simulink model "walkingRobotRL3D"  (R2020b)
settings: Solver=ode23t  StartTime=0.0  StopTime=Tf  RelTol=1e-2  EnableMultiTasking=on
PreLoadFcn:
  | robotParametersRL
undefined symbols (not defined in the file): agent, ankleD_pitch_jointMAX, ankleD_pitch_jointMIN, ankleD_roll_jointMAX, ankleD_roll_jointMIN, ankleI_pitch_jointMAX, ankleI_pitch_jointMIN, ankleI_roll_jointMAX, ankleI_roll_jointMIN, getSampleTime, height_plane, hipD_pitch_jointMAX, hipD_pitch_jointMIN, hipD_roll_jointMAX, hipD_roll_jointMIN, hipI_pitch_jointMAX, hipI_pitch_jointMIN, hipI_roll_jointMAX, hipI_roll_jointMIN, init_angs_L, init_angs_R, init_height, joint_damping, joint_limit_damping, joint_limit_stiffness, joint_stiffness, kneeD_jointMAX, kneeD_jointMIN, kneeI_jointMAX, kneeI_jointMIN, lower_leg_I0, lower_leg_length, lower_leg_mass, lower_leg_x, lower_leg_y, muscle_nominal_length, p10_ankleD_roll, plane_x, plane_y, regulator_type, tau, Tf, torso_height, torso_length, torso_offset_x, torso_offset_z, torso_width, torso_x, torso_y, torso_z, Ts, upper_leg_I0, upper_leg_length, upper_leg_mass, upper_leg_x, upper_leg_y, v10_ankleD_pitch, v10_ankleD_roll, v10_ankleI_pitch, v10_ankleI_roll ... (+41)
libraries: sm_lib x222, simulink x183, nesl_utility x130, walkingRobotUtils x69, rllib x2
(part 14 of 24)

== system walkingRobotRL3D/Walking Robot (Angle based)/Antagonistic PAM Right Leg/ankleD_pitch PAM/Spring and damping model ==
  F1 : Inport
  F2 : Inport  Port=2
  P1 : Inport  Port=3
  P2 : Inport  Port=4
  Bar->kPa : Gain  Gain=100
  Bar->kPa1 : Gain  Gain=100
  Dynamic muscle 2 : Subsystem
  Dynamics muscle 1 : Subsystem
  Fplot : Scope  NumInputPorts=2
  Pplot : Scope  NumInputPorts=2
  Rplot : Scope  NumInputPorts=2
  Splot : Scope  NumInputPorts=2
  Stimation of spring coefficients : MATLAB Function  TreatAsAtomicUnit=on
  Stimation of spring coefficients1 : MATLAB Function  TreatAsAtomicUnit=on
  Unit Delay{,1..3} (4 alike) : UnitDelay  SampleTime=-1  HasFrameUpgradeWarning=on
  getDeltaXmax : Subsystem
  getDeltaXmax1 : Subsystem
  x(%)->x(m) : Gain  Gain=muscle_nominal_length/100
  x(%)->x(m)1 : Gain  Gain=muscle_nominal_length/100
  x1(m)->x1(%) : Gain  Gain=100/muscle_nominal_length
  x2(m)->x2(%) : Gain  Gain=100/muscle_nominal_length
  xplot : Scope  NumInputPorts=2
  x1 : Outport
  x2 : Outport  Port=2
  wires:
  Dynamics muscle 1/1(R1) -> Unit Delay/1, Unit Delay2/1
  Dynamic muscle 2/1(R2) -> Unit Delay1/1, Unit Delay3/1
  F1/1 -> Stimation of spring coefficients/4(F1), Fplot/1, Dynamics muscle 1/1(F1)
  Dynamic muscle 2/2(x2) -> x2(m)->x2(%)/1
  Dynamics muscle 1/2(x1) -> x1(m)->x1(%)/1
  P1/1 -> Pplot/1, Bar->kPa/1
  Bar->kPa/1 -> Stimation of spring coefficients/1(P1), getDeltaXmax/1(In1)
  P2/1 -> Pplot/2, Bar->kPa1/1
  Bar->kPa1/1 -> getDeltaXmax1/1(In1), Stimation of spring coefficients1/2(P2)
  Stimation of spring coefficients/1(S1) -> Splot/1, Dynamics muscle 1/2(S1)
  Stimation of spring coefficients1/1(S2) -> Splot/2, Dynamic muscle 2/1(S2)
  getDeltaXmax/1(dmax1) -> Stimation of spring coefficients/5(dmax1_per), x(%)->x(m)/1
  x(%)->x(m)/1 -> Stimation of spring coefficients/3(dmax1)
  getDeltaXmax1/1(dmax2) -> Stimation of spring coefficients1/5(dmax2_per), x(%)->x(m)1/1
  x(%)->x(m)1/1 -> Stimation of spring coefficients1/4(dmax2)
  x2(m)->x2(%)/1 -> xplot/2, x2/1
  x1(m)->x1(%)/1 -> xplot/1, x1/1
  F2/1 -> Stimation of spring coefficients1/1(F2), Fplot/2, Dynamic muscle 2/3(F2)
  Unit Delay/1 -> Stimation of spring coefficients1/3(Fload)
  Unit Delay1/1 -> Stimation of spring coefficients/2(Fload)
  Unit Delay2/1 -> Rplot/1, Dynamic muscle 2/2(R1)
  Unit Delay3/1 -> Rplot/2, Dynamics muscle 1/3(R2)

== system walkingRobotRL3D/Walking Robot (Angle based)/Antagonistic PAM Right Leg/ankleD_roll PAM/Spring and damping model ==
  F1 : Inport
  F2 : Inport  Port=2
  P1 : Inport  Port=3
  P2 : Inport  Port=4
  Bar->kPa : Gain  Gain=100
  Bar->kPa1 : Gain  Gain=100
  Dynamic muscle 2 : Subsystem
  Dynamics muscle 1 : Subsystem
  Fplot : Scope  NumInputPorts=2
  Pplot : Scope  NumInputPorts=2
  Rplot : Scope  NumInputPorts=2
  Splot : Scope  NumInputPorts=2
  Stimation of spring coefficients : MATLAB Function  TreatAsAtomicUnit=on
  Stimation of spring coefficients1 : MATLAB Function  TreatAsAtomicUnit=on
  Unit Delay{,1..3} (4 alike) : UnitDelay  SampleTime=-1  HasFrameUpgradeWarning=on
  getDeltaXmax : Subsystem
  getDeltaXmax1 : Subsystem
  x(%)->x(m) : Gain  Gain=muscle_nominal_length/100
  x(%)->x(m)1 : Gain  Gain=muscle_nominal_length/100
  x1(m)->x1(%) : Gain  Gain=100/muscle_nominal_length
  x2(m)->x2(%) : Gain  Gain=100/muscle_nominal_length
  xplot : Scope  NumInputPorts=2
  x1 : Outport
  x2 : Outport  Port=2
  wires:
  Dynamics muscle 1/1(R1) -> Unit Delay/1, Unit Delay2/1
  Dynamic muscle 2/1(R2) -> Unit Delay1/1, Unit Delay3/1
  F1/1 -> Stimation of spring coefficients/4(F1), Fplot/1, Dynamics muscle 1/1(F1)
  Dynamic muscle 2/2(x2) -> x2(m)->x2(%)/1
  Dynamics muscle 1/2(x1) -> x1(m)->x1(%)/1
  P1/1 -> Pplot/1, Bar->kPa/1
  Bar->kPa/1 -> Stimation of spring coefficients/1(P1), getDeltaXmax/1(In1)
  P2/1 -> Pplot/2, Bar->kPa1/1
  Bar->kPa1/1 -> getDeltaXmax1/1(In1), Stimation of spring coefficients1/2(P2)
  Stimation of spring coefficients/1(S1) -> Splot/1, Dynamics muscle 1/2(S1)
  Stimation of spring coefficients1/1(S2) -> Splot/2, Dynamic muscle 2/1(S2)
  getDeltaXmax/1(dmax1) -> Stimation of spring coefficients/5(dmax1_per), x(%)->x(m)/1
  x(%)->x(m)/1 -> Stimation of spring coefficients/3(dmax1)
  getDeltaXmax1/1(dmax2) -> Stimation of spring coefficients1/5(dmax2_per), x(%)->x(m)1/1
  x(%)->x(m)1/1 -> Stimation of spring coefficients1/4(dmax2)
  x2(m)->x2(%)/1 -> xplot/2, x2/1
  x1(m)->x1(%)/1 -> xplot/1, x1/1
  F2/1 -> Stimation of spring coefficients1/1(F2), Fplot/2, Dynamic muscle 2/3(F2)
  Unit Delay/1 -> Stimation of spring coefficients1/3(Fload)
  Unit Delay1/1 -> Stimation of spring coefficients/2(Fload)
  Unit Delay2/1 -> Rplot/1, Dynamic muscle 2/2(R1)
  Unit Delay3/1 -> Rplot/2, Dynamics muscle 1/3(R2)

== system walkingRobotRL3D/Walking Robot (Angle based)/Antagonistic PAM Right Leg/hipD_pitch PAM/Spring and damping model ==
  F1 : Inport
  F2 : Inport  Port=2
  P1 : Inport  Port=3
  P2 : Inport  Port=4
  Bar->kPa : Gain  Gain=100
  Bar->kPa1 : Gain  Gain=100
  Dynamic muscle 2 : Subsystem
  Dynamics muscle 1 : Subsystem
  Fplot : Scope  NumInputPorts=2
  Pplot : Scope  NumInputPorts=2
  Rplot : Scope  NumInputPorts=2
  Splot : Scope  NumInputPorts=2
  Stimation of spring coefficients : MATLAB Function  TreatAsAtomicUnit=on
  Stimation of spring coefficients1 : MATLAB Function  TreatAsAtomicUnit=on
  Unit Delay{,1..3} (4 alike) : UnitDelay  SampleTime=-1  HasFrameUpgradeWarning=on
  getDeltaXmax : Subsystem
  getDeltaXmax1 : Subsystem
  x(%)->x(m) : Gain  Gain=muscle_nominal_length/100
  x(%)->x(m)1 : Gain  Gain=muscle_nominal_length/100
  x1(m)->x1(%) : Gain  Gain=100/muscle_nominal_length
  x2(m)->x2(%) : Gain  Gain=100/muscle_nominal_length
  xplot : Scope  NumInputPorts=2
  x1 : Outport
  x2 : Outport  Port=2
  wires:
  Dynamics muscle 1/1(R1) -> Unit Delay/1, Unit Delay2/1
  Dynamic muscle 2/1(R2) -> Unit Delay1/1, Unit Delay3/1
  F1/1 -> Stimation of spring coefficients/4(F1), Fplot/1, Dynamics muscle 1/1(F1)
  Dynamic muscle 2/2(x2) -> x2(m)->x2(%)/1
  Dynamics muscle 1/2(x1) -> x1(m)->x1(%)/1
  P1/1 -> Pplot/1, Bar->kPa/1
  Bar->kPa/1 -> Stimation of spring coefficients/1(P1), getDeltaXmax/1(In1)
  P2/1 -> Pplot/2, Bar->kPa1/1
  Bar->kPa1/1 -> getDeltaXmax1/1(In1), Stimation of spring coefficients1/2(P2)
  Stimation of spring coefficients/1(S1) -> Splot/1, Dynamics muscle 1/2(S1)
  Stimation of spring coefficients1/1(S2) -> Splot/2, Dynamic muscle 2/1(S2)
  getDeltaXmax/1(dmax1) -> Stimation of spring coefficients/5(dmax1_per), x(%)->x(m)/1
  x(%)->x(m)/1 -> Stimation of spring coefficients/3(dmax1)
  getDeltaXmax1/1(dmax2) -> Stimation of spring coefficients1/5(dmax2_per), x(%)->x(m)1/1
  x(%)->x(m)1/1 -> Stimation of spring coefficients1/4(dmax2)
  x2(m)->x2(%)/1 -> xplot/2, x2/1
  x1(m)->x1(%)/1 -> xplot/1, x1/1
  F2/1 -> Stimation of spring coefficients1/1(F2), Fplot/2, Dynamic muscle 2/3(F2)
  Unit Delay/1 -> Stimation of spring coefficients1/3(Fload)
  Unit Delay1/1 -> Stimation of spring coefficients/2(Fload)
  Unit Delay2/1 -> Rplot/1, Dynamic muscle 2/2(R1)
  Unit Delay3/1 -> Rplot/2, Dynamics muscle 1/3(R2)

== system walkingRobotRL3D/Walking Robot (Angle based)/Antagonistic PAM Right Leg/hipD_roll PAM/Spring and damping model ==
  F1 : Inport
  F2 : Inport  Port=2
  P1 : Inport  Port=3
  P2 : Inport  Port=4
  Bar->kPa : Gain  Gain=100
  Bar->kPa1 : Gain  Gain=100
  Dynamic muscle 2 : Subsystem
  Dynamics muscle 1 : Subsystem
  Fplot : Scope  NumInputPorts=2
  Pplot : Scope  NumInputPorts=2
  Rplot : Scope  NumInputPorts=2
  Splot : Scope  NumInputPorts=2
  Stimation of spring coefficients : MATLAB Function  TreatAsAtomicUnit=on
  Stimation of spring coefficients1 : MATLAB Function  TreatAsAtomicUnit=on
  Unit Delay{,1..3} (4 alike) : UnitDelay  SampleTime=-1  HasFrameUpgradeWarning=on
  getDeltaXmax : Subsystem
  getDeltaXmax1 : Subsystem
  x(%)->x(m) : Gain  Gain=muscle_nominal_length/100
  x(%)->x(m)1 : Gain  Gain=muscle_nominal_length/100
  x1(m)->x1(%) : Gain  Gain=100/muscle_nominal_length
  x2(m)->x2(%) : Gain  Gain=100/muscle_nominal_length
  xplot : Scope  NumInputPorts=2
  x1 : Outport
  x2 : Outport  Port=2
  wires:
  Dynamics muscle 1/1(R1) -> Unit Delay/1, Unit Delay2/1
  Dynamic muscle 2/1(R2) -> Unit Delay1/1, Unit Delay3/1
  F1/1 -> Stimation of spring coefficients/4(F1), Fplot/1, Dynamics muscle 1/1(F1)
  Dynamic muscle 2/2(x2) -> x2(m)->x2(%)/1
  Dynamics muscle 1/2(x1) -> x1(m)->x1(%)/1
  P1/1 -> Pplot/1, Bar->kPa/1
  Bar->kPa/1 -> Stimation of spring coefficients/1(P1), getDeltaXmax/1(In1)
  P2/1 -> Pplot/2, Bar->kPa1/1
  Bar->kPa1/1 -> getDeltaXmax1/1(In1), Stimation of spring coefficients1/2(P2)
  Stimation of spring coefficients/1(S1) -> Splot/1, Dynamics muscle 1/2(S1)
  Stimation of spring coefficients1/1(S2) -> Splot/2, Dynamic muscle 2/1(S2)
  getDeltaXmax/1(dmax1) -> Stimation of spring coefficients/5(dmax1_per), x(%)->x(m)/1
  x(%)->x(m)/1 -> Stimation of spring coefficients/3(dmax1)
  getDeltaXmax1/1(dmax2) -> Stimation of spring coefficients1/5(dmax2_per), x(%)->x(m)1/1
  x(%)->x(m)1/1 -> Stimation of spring coefficients1/4(dmax2)
  x2(m)->x2(%)/1 -> xplot/2, x2/1
  x1(m)->x1(%)/1 -> xplot/1, x1/1
  F2/1 -> Stimation of spring coefficients1/1(F2), Fplot/2, Dynamic muscle 2/3(F2)
  Unit Delay/1 -> Stimation of spring coefficients1/3(Fload)
  Unit Delay1/1 -> Stimation of spring coefficients/2(Fload)
  Unit Delay2/1 -> Rplot/1, Dynamic muscle 2/2(R1)
  Unit Delay3/1 -> Rplot/2, Dynamics muscle 1/3(R2)

== system walkingRobotRL3D/Walking Robot (Angle based)/Antagonistic PAM Right Leg/kneeD PAM/Spring and damping model ==
  F1 : Inport
  F2 : Inport  Port=2
  P1 : Inport  Port=3
  P2 : Inport  Port=4
  Bar->kPa : Gain  Gain=100
  Bar->kPa1 : Gain  Gain=100
  Dynamic muscle 2 : Subsystem
  Dynamics muscle 1 : Subsystem
  Fplot : Scope  NumInputPorts=2
  Pplot : Scope  NumInputPorts=2
  Rplot : Scope  NumInputPorts=2
  Splot : Scope  NumInputPorts=2
  Stimation of spring coefficients : MATLAB Function  TreatAsAtomicUnit=on
  Stimation of spring coefficients1 : MATLAB Function  TreatAsAtomicUnit=on
  Unit Delay{,1..3} (4 alike) : UnitDelay  SampleTime=-1  HasFrameUpgradeWarning=on
  getDeltaXmax : Subsystem
  getDeltaXmax1 : Subsystem
  x(%)->x(m) : Gain  Gain=muscle_nominal_length/100
  x(%)->x(m)1 : Gain  Gain=muscle_nominal_length/100
  x1(m)->x1(%) : Gain  Gain=100/muscle_nominal_length
  x2(m)->x2(%) : Gain  Gain=100/muscle_nominal_length
  xplot : Scope  NumInputPorts=2
  x1 : Outport
  x2 : Outport  Port=2
  wires:
  Dynamics muscle 1/1(R1) -> Unit Delay/1, Unit Delay2/1
  Dynamic muscle 2/1(R2) -> Unit Delay1/1, Unit Delay3/1
  F1/1 -> Stimation of spring coefficients/4(F1), Fplot/1, Dynamics muscle 1/1(F1)
  Dynamic muscle 2/2(x2) -> x2(m)->x2(%)/1
  Dynamics muscle 1/2(x1) -> x1(m)->x1(%)/1
  P1/1 -> Pplot/1, Bar->kPa/1
  Bar->kPa/1 -> Stimation of spring coefficients/1(P1), getDeltaXmax/1(In1)
  P2/1 -> Pplot/2, Bar->kPa1/1
  Bar->kPa1/1 -> getDeltaXmax1/1(In1), Stimation of spring coefficients1/2(P2)
  Stimation of spring coefficients/1(S1) -> Splot/1, Dynamics muscle 1/2(S1)
  Stimation of spring coefficients1/1(S2) -> Splot/2, Dynamic muscle 2/1(S2)
  getDeltaXmax/1(dmax1) -> Stimation of spring coefficients/5(dmax1_per), x(%)->x(m)/1
  x(%)->x(m)/1 -> Stimation of spring coefficients/3(dmax1)
  getDeltaXmax1/1(dmax2) -> Stimation of spring coefficients1/5(dmax2_per), x(%)->x(m)1/1
  x(%)->x(m)1/1 -> Stimation of spring coefficients1/4(dmax2)
  x2(m)->x2(%)/1 -> xplot/2, x2/1
  x1(m)->x1(%)/1 -> xplot/1, x1/1
  F2/1 -> Stimation of spring coefficients1/1(F2), Fplot/2, Dynamic muscle 2/3(F2)
  Unit Delay/1 -> Stimation of spring coefficients1/3(Fload)
  Unit Delay1/1 -> Stimation of spring coefficients/2(Fload)
  Unit Delay2/1 -> Rplot/1, Dynamic muscle 2/2(R1)
  Unit Delay3/1 -> Rplot/2, Dynamics muscle 1/3(R2)

== system walkingRobotRL3D/Walking Robot (Angle based)/Dynamic model of antagonistic PAM actuators/Spring//Damping (Muscles 1)/Get_delta_xmax1 ==
  P1 : Inport
  Bar->kPa : Product
  Constant : Constant  Value=100
  Demux : Demux  Outputs=10
  Mux : Mux  Inputs=10
  Mux1 : Mux  Inputs=10
  getDeltaXmax : Subsystem
  getDeltaXmax1 : Subsystem
  getDeltaXmax2 : Subsystem
  getDeltaXmax3 : Subsystem
  getDeltaXmax4 : Subsystem
  getDeltaXmax5 : Subsystem
  getDeltaXmax6 : Subsystem
  getDeltaXmax7 : Subsystem
  getDeltaXmax8 : Subsystem
  getDeltaXmax9 : Subsystem
  xmax_muscles1 : Outport
  delta_xmax_muscles1_per : Outport  Port=2
  wires:
  P1/1 -> Bar->kPa/2
  Bar->kPa/1 -> Demux/1
  Constant/1 -> Bar->kPa/1
  Mux/1 -> xmax_muscles1/1
  Demux/1 -> getDeltaXmax/1(In1)
  getDeltaXmax/1(Out1) -> Mux/1
  Mux1/1 -> delta_xmax_muscles1_per/1
  Demux/2 -> getDeltaXmax1/1(In1)
  Demux/3 -> getDeltaXmax2/1(In1)
  Demux/4 -> getDeltaXmax3/1(In1)
  Demux/5 -> getDeltaXmax4/1(In1)
  Demux/6 -> getDeltaXmax5/1(In1)
  Demux/7 -> getDeltaXmax6/1(In1)
  Demux/8 -> getDeltaXmax7/1(In1)
  Demux/9 -> getDeltaXmax8/1(In1)
  getDeltaXmax1/1(Out1) -> Mux/2
  getDeltaXmax2/1(Out1) -> Mux/3
  getDeltaXmax3/1(Out1) -> Mux/4
  getDeltaXmax4/1(Out1) -> Mux/5
  getDeltaXmax5/1(Out1) -> Mux/6
  getDeltaXmax6/1(Out1) -> Mux/7
  getDeltaXmax7/1(Out1) -> Mux/8
  getDeltaXmax8/1(Out1) -> Mux/9
  getDeltaXmax9/1(Out1) -> Mux/10
  getDeltaXmax/2(Out2) -> Mux1/1
  getDeltaXmax1/2(Out2) -> Mux1/2
  getDeltaXmax2/2(Out2) -> Mux1/3
  getDeltaXmax3/2(Out2) -> Mux1/4
  getDeltaXmax4/2(Out2) -> Mux1/5
  getDeltaXmax5/2(Out2) -> Mux1/6
  getDeltaXmax6/2(Out2) -> Mux1/7
  getDeltaXmax7/2(Out2) -> Mux1/8
  getDeltaXmax8/2(Out2) -> Mux1/9
  Demux/10 -> getDeltaXmax9/1(In1)
  getDeltaXmax9/2(Out2) -> Mux1/10

== system walkingRobotRL3D/Walking Robot (Angle based)/Dynamic model of antagonistic PAM actuators/Spring//Damping (Muscles 1)/Get_x1_ankleD_pitch ==
  F1_ankleD_pitchl : Inport
  F2_ankleD_pitch : Inport  Port=2
  S_coef : Inport  Port=3
  Add : Sum  Inputs=+--
  Constant : Constant  Value=tau
  Constant1 : Constant
  Constant2 : Constant  Commented=on  Value=-3.9322
  D_coef : Product
  Divide : Product  Inputs=*/
  IC : InitialCondition  Commented=through  Value=10000
  Integrator : Integrator  InitialCondition=x10_ankleD_pitch
  To Workspace : ToWorkspace  VariableName=S1_ankleD_pitch  SaveFormat=Timeseries  SampleTime=-1
  To Workspace1 : ToWorkspace  VariableName=D1_ankleD_pitch  SaveFormat=Timeseries  SampleTime=-1
  x./D : Product
  xS : Product
  x1_ankleD_pitch : Outport
  wires:
  xS/1 -> Add/3
  x./D/1 -> Integrator/1
  Constant/1 -> D_coef/1
  Divide/1 -> x./D/1
  Constant1/1 -> Divide/1
  D_coef/1 -> To Workspace1/1, Divide/2
  Integrator/1 -> x1_ankleD_pitch/1, xS/1
  IC/1 -> xS/2, To Workspace/1, D_coef/2
  F1_ankleD_pitchl/1 -> Add/1
  F2_ankleD_pitch/1 -> Add/2
  S_coef/1 -> IC/1
  Add/1 -> x./D/2

== system walkingRobotRL3D/Walking Robot (Angle based)/Dynamic model of antagonistic PAM actuators/Spring//Damping (Muscles 1)/Get_x1_ankleD_roll ==
  F1_ankleD_roll : Inport
  F2_ankleD_roll : Inport  Port=2
  S_coef : Inport  Port=3
  Add : Sum  Inputs=+--
  Constant : Constant  Value=tau
  Constant1 : Constant
  Constant2 : Constant  Commented=on  Value=-3.9322
  D_coef : Product
  Divide : Product  Inputs=*/
  IC : InitialCondition  Commented=through  Value=10000
  Integrator : Integrator  InitialCondition=x10_ankleD_roll
  To Workspace : ToWorkspace  VariableName=S1_ankleD_roll  SaveFormat=Timeseries  SampleTime=-1
  To Workspace1 : ToWorkspace  VariableName=D1_ankleD_roll  SaveFormat=Timeseries  SampleTime=-1
  x./D : Product
  xS : Product
  x1_ankleD_roll : Outport
  wires:
  xS/1 -> Add/3
  x./D/1 -> Integrator/1
  Constant/1 -> D_coef/1
  Divide/1 -> x./D/1
  Constant1/1 -> Divide/1
  D_coef/1 -> To Workspace1/1, Divide/2
  Integrator/1 -> x1_ankleD_roll/1, xS/1
  IC/1 -> xS/2, To Workspace/1, D_coef/2
  F1_ankleD_roll/1 -> Add/1
  F2_ankleD_roll/1 -> Add/2
  Add/1 -> x./D/2
  S_coef/1 -> IC/1

== system walkingRobotRL3D/Walking Robot (Angle based)/Dynamic model of antagonistic PAM actuators/Spring//Damping (Muscles 1)/Get_x1_ankleI_pitch ==
  F1_ankleI_pitch : Inport
  F2_ankleI_pitch : Inport  Port=2
  S_coef : Inport  Port=3
  Add : Sum  Inputs=+--
  Constant : Constant  Value=tau
  Constant1 : Constant
  D_coef : Product
  Divide : Product  Inputs=*/
  Integrator : Integrator  InitialCondition=x10_ankleI_pitch
  x./D : Product
  xS : Product
  x1_ankleI_pitch : Outport
  wires:
  xS/1 -> Add/3
  Add/1 -> x./D/2
  F1_ankleI_pitch/1 -> Add/1
  F2_ankleI_pitch/1 -> Add/2
  Integrator/1 -> x1_ankleI_pitch/1, xS/1
  S_coef/1 -> D_coef/2, xS/2
  x./D/1 -> Integrator/1
  Constant/1 -> D_coef/1
  Divide/1 -> x./D/1
  Constant1/1 -> Divide/1
  D_coef/1 -> Divide/2

== system walkingRobotRL3D/Walking Robot (Angle based)/Dynamic model of antagonistic PAM actuators/Spring//Damping (Muscles 1)/Get_x1_ankleI_roll ==
  F1_ankleI_roll : Inport
  F2_ankleI_roll : Inport  Port=2
  S_coef : Inport  Port=3
  Add : Sum  Inputs=+--
  Constant : Constant  Value=tau
  Constant1 : Constant
  D_coef : Product
  Divide : Product  Inputs=*/
  Integrator : Integrator  InitialCondition=x10_ankleI_roll
  x./D : Product
  xS : Product
  x1_ankleI_roll : Outport
  wires:
  xS/1 -> Add/3
  Add/1 -> x./D/2
  F1_ankleI_roll/1 -> Add/1
  F2_ankleI_roll/1 -> Add/2
  Integrator/1 -> x1_ankleI_roll/1, xS/1
  S_coef/1 -> D_coef/2, xS/2
  x./D/1 -> Integrator/1
  Constant/1 -> D_coef/1
  Divide/1 -> x./D/1
  Constant1/1 -> Divide/1
  D_coef/1 -> Divide/2

== system walkingRobotRL3D/Walking Robot (Angle based)/Dynamic model of antagonistic PAM actuators/Spring//Damping (Muscles 1)/Get_x1_hipD_pitch ==
  F1_hipD_pitch : Inport
  F2_hipD_pitch : Inport  Port=2
  S_coef : Inport  Port=3
  Add : Sum  Inputs=+--
  Constant : Constant  Value=tau
  Constant1 : Constant
  D_coef : Product
  Divide : Product  Inputs=*/
  Integrator : Integrator  InitialCondition=x10_hipD_pitch
  x./D : Product
  xS : Product
  x1_hipD_pitch : Outport
  wires:
  xS/1 -> Add/3
  Add/1 -> x./D/2
  F1_hipD_pitch/1 -> Add/1
  F2_hipD_pitch/1 -> Add/2
  Integrator/1 -> x1_hipD_pitch/1, xS/1
  S_coef/1 -> D_coef/2, xS/2
  x./D/1 -> Integrator/1
  Constant/1 -> D_coef/1
  Divide/1 -> x./D/1
  Constant1/1 -> Divide/1
  D_coef/1 -> Divide/2

== system walkingRobotRL3D/Walking Robot (Angle based)/Dynamic model of antagonistic PAM actuators/Spring//Damping (Muscles 1)/Get_x1_hipD_roll ==
  F1_hipD_roll : Inport
  F2_hipD_roll : Inport  Port=2
  S_coef : Inport  Port=3
  Add : Sum  Inputs=+--
  Constant : Constant  Value=tau
  Constant1 : Constant
  D_coef : Product
  Divide : Product  Inputs=*/
  Integrator : Integrator  InitialCondition=x10_hipD_roll
  x./D : Product
  xS : Product
  x1_hipD_roll : Outport
  wires:
  xS/1 -> Add/3
  Add/1 -> x./D/2
  F1_hipD_roll/1 -> Add/1
  F2_hipD_roll/1 -> Add/2
  Integrator/1 -> x1_hipD_roll/1, xS/1
  S_coef/1 -> D_coef/2, xS/2
  x./D/1 -> Integrator/1
  Constant/1 -> D_coef/1
  Divide/1 -> x./D/1
  Constant1/1 -> Divide/1
  D_coef/1 -> Divide/2

== system walkingRobotRL3D/Walking Robot (Angle based)/Dynamic model of antagonistic PAM actuators/Spring//Damping (Muscles 1)/Get_x1_hipI_pitch ==
  F1_hipI_pitch : Inport
  F2_hipI_pitch : Inport  Port=2
  S_coef : Inport  Port=3
  Add : Sum  Inputs=+--
  Constant : Constant  Value=tau
  Constant1 : Constant
  D_coef : Product
  Divide : Product  Inputs=*/
  Integrator : Integrator  InitialCondition=x10_hipI_pitch
  Relay : Relay  Commented=through  OnSwitchValue=28.12*muscle_nominal_length/100  OffSwitchValue=0  OnOutputValue=28.12*muscle_nominal_length/100
  x./D : Product
  xS : Product
  x1_hipI_pitch : Outport
  wires:
  xS/1 -> Add/3
  Add/1 -> x./D/2
  F1_hipI_pitch/1 -> Add/1
  F2_hipI_pitch/1 -> Add/2
  S_coef/1 -> D_coef/2, xS/2
  x./D/1 -> Integrator/1
  Constant/1 -> D_coef/1
  Divide/1 -> x./D/1
  Constant1/1 -> Divide/1
  D_coef/1 -> Divide/2
  Integrator/1 -> Relay/1
  Relay/1 -> xS/1, x1_hipI_pitch/1

== system walkingRobotRL3D/Walking Robot (Angle based)/Dynamic model of antagonistic PAM actuators/Spring//Damping (Muscles 1)/Get_x1_hipI_roll ==
  F1_hipI_roll : Inport
  F2_hipI_roll : Inport  Port=2
  S_coef : Inport  Port=3
  Add : Sum  Inputs=+--
  Constant : Constant  Value=tau
  Constant1 : Constant
  D_coef : Product
  Divide : Product  Inputs=*/
  Integrator : Integrator  InitialCondition=x10_hipI_roll
  x./D : Product
  xS : Product
  x1_hipI_roll : Outport
  wires:
  xS/1 -> Add/3
  Add/1 -> x./D/2
  F1_hipI_roll/1 -> Add/1
  F2_hipI_roll/1 -> Add/2
  Integrator/1 -> x1_hipI_roll/1, xS/1
  S_coef/1 -> D_coef/2, xS/2
  x./D/1 -> Integrator/1
  Constant/1 -> D_coef/1
  Divide/1 -> x./D/1
  Constant1/1 -> Divide/1
  D_coef/1 -> Divide/2

== system walkingRobotRL3D/Walking Robot (Angle based)/Dynamic model of antagonistic PAM actuators/Spring//Damping (Muscles 1)/Get_x1_kneeD_1 ==
  F1_kneeD : Inport
  F2_kneeD : Inport  Port=2
  S_coef : Inport  Port=3
  Add : Sum  Inputs=++-
  Constant : Constant  Value=tau
  Constant1 : Constant
  D_coef : Product
  Divide : Product  Inputs=*/
  Integrator : Integrator  InitialCondition=x10_kneeD
  x./D : Product
  xS : Product
  x1_kneeD : Outport
  wires:
  xS/1 -> Add/3
  Add/1 -> x./D/2
  F1_kneeD/1 -> Add/1
  F2_kneeD/1 -> Add/2
  Integrator/1 -> x1_kneeD/1, xS/1
  S_coef/1 -> D_coef/2, xS/2
  x./D/1 -> Integrator/1
  Constant/1 -> D_coef/1
  Divide/1 -> x./D/1
  Constant1/1 -> Divide/1
  D_coef/1 -> Divide/2

== system walkingRobotRL3D/Walking Robot (Angle based)/Dynamic model of antagonistic PAM actuators/Spring//Damping (Muscles 1)/Get_x1_kneeI ==
  F1_kneeI : Inport
  F2_kneeI : Inport  Port=2
  S_coef : Inport  Port=3
  Abs2 : Abs
  Add : Sum  Inputs=++-
  Constant : Constant  Value=tau
  Constant1 : Constant
  D_coef : Product
  Divide : Product  Inputs=*/
  Integrator : Integrator  InitialCondition=x10_kneeI
  x./D : Product
  xS : Product
  x1_kneeI : Outport
  wires:
  F1_kneeI/1 -> Add/1
  Integrator/1 -> x1_kneeI/1, xS/1
  S_coef/1 -> Abs2/1
  x./D/1 -> Integrator/1
  Constant/1 -> D_coef/1
  Divide/1 -> x./D/1
  Constant1/1 -> Divide/1
  D_coef/1 -> Divide/2
  Abs2/1 -> xS/2, D_coef/2
  xS/1 -> Add/3
  F2_kneeI/1 -> Add/2
  Add/1 -> x./D/2

== system walkingRobotRL3D/Walking Robot (Angle based)/Dynamic model of antagonistic PAM actuators/Spring//Damping (Muscles 2)/Get_x2_ankleD_pitch ==
  F1_ankleD_pitch : Inport
  F2_ankleD_pitch : Inport  Port=2
  S2_coef : Inport  Port=3
  Add : Sum  Inputs=-+-
  Constant : Constant  Value=tau
  Constant1 : Constant
  Constant2 : Constant  Commented=on  Value=3.9338
  D_coef : Product
  Divide : Product  Inputs=*/
  IC : InitialCondition  Commented=through  Value=3.9338
  Integrator : Integrator  InitialCondition=x20_ankleD_pitch
  To Workspace : ToWorkspace  VariableName=S2_ankleD_pitch  SaveFormat=Timeseries  SampleTime=-1
  x./D : Product
  xS : Product
  x2_ankleD_pitch : Outport
  wires:
  xS/1 -> Add/3
  Add/1 -> x./D/2
  F1_ankleD_pitch/1 -> Add/1
  F2_ankleD_pitch/1 -> Add/2
  Integrator/1 -> x2_ankleD_pitch/1, xS/1
  x./D/1 -> Integrator/1
  Constant/1 -> D_coef/1
  Divide/1 -> x./D/1
  Constant1/1 -> Divide/1
  IC/1 -> To Workspace/1, D_coef/2, xS/2
  D_coef/1 -> Divide/2
  S2_coef/1 -> IC/1

== system walkingRobotRL3D/Walking Robot (Angle based)/Dynamic model of antagonistic PAM actuators/Spring//Damping (Muscles 2)/Get_x2_ankleD_roll ==
  F1_ankleD_roll : Inport
  F2_ankleD_roll : Inport  Port=2
  S2_coef : Inport  Port=3
  Add : Sum  Inputs=-+-
  Constant : Constant  Value=tau
  Constant1 : Constant
  Constant2 : Constant  Commented=on  Value=3.9338
  D_coef : Product
  Divide : Product  Inputs=*/
  IC : InitialCondition  Commented=through  Value=3.9338
  Integrator : Integrator  InitialCondition=x20_ankleD_roll
  To Workspace : ToWorkspace  VariableName=S2_ankleD_roll  SaveFormat=Timeseries  SampleTime=-1
  x./D : Product
  xS : Product
  x2_ankleD_roll : Outport
  wires:
  xS/1 -> Add/3
  Add/1 -> x./D/2
  F1_ankleD_roll/1 -> Add/1
  F2_ankleD_roll/1 -> Add/2
  Integrator/1 -> x2_ankleD_roll/1, xS/1
  x./D/1 -> Integrator/1
  Constant/1 -> D_coef/1
  Divide/1 -> x./D/1
  Constant1/1 -> Divide/1
  IC/1 -> To Workspace/1, D_coef/2, xS/2
  D_coef/1 -> Divide/2
  S2_coef/1 -> IC/1

== system walkingRobotRL3D/Walking Robot (Angle based)/Dynamic model of antagonistic PAM actuators/Spring//Damping (Muscles 2)/Get_x2_ankleI_pitch ==
  F1_ankleI_pitch : Inport
  F2_ankleI_pitch : Inport  Port=2
  S2_coef : Inport  Port=3
  Add : Sum  Inputs=-+-
  Constant : Constant  Value=tau
  Constant1 : Constant
  D_coef : Product
  Divide : Product  Inputs=*/
  Integrator : Integrator  InitialCondition=x20_ankleI_pitch
  x./D : Product
  xS : Product
  x2_ankleI_pitch : Outport
  wires:
  xS/1 -> Add/3
  Add/1 -> x./D/2
  F1_ankleI_pitch/1 -> Add/1
  F2_ankleI_pitch/1 -> Add/2
  Integrator/1 -> x2_ankleI_pitch/1, xS/1
  S2_coef/1 -> D_coef/2, xS/2
  x./D/1 -> Integrator/1
  Constant/1 -> D_coef/1
  Divide/1 -> x./D/1
  Constant1/1 -> Divide/1
  D_coef/1 -> Divide/2

== system walkingRobotRL3D/Walking Robot (Angle based)/Dynamic model of antagonistic PAM actuators/Spring//Damping (Muscles 2)/Get_x2_ankleI_roll ==
  F1_ankleI_roll : Inport
  F2_ankleI_roll : Inport  Port=2
  S2_coef : Inport  Port=3
  Add : Sum  Inputs=-+-
  Constant : Constant  Value=tau
  Constant1 : Constant
  D_coef : Product
  Divide : Product  Inputs=*/
  Integrator : Integrator  InitialCondition=x20_ankleI_roll
  x./D : Product
  xS : Product
  x2_ankleI_roll : Outport
  wires:
  xS/1 -> Add/3
  Add/1 -> x./D/2
  F1_ankleI_roll/1 -> Add/1
  F2_ankleI_roll/1 -> Add/2
  Integrator/1 -> x2_ankleI_roll/1, xS/1
  S2_coef/1 -> D_coef/2, xS/2
  x./D/1 -> Integrator/1
  Constant/1 -> D_coef/1
  Divide/1 -> x./D/1
  Constant1/1 -> Divide/1
  D_coef/1 -> Divide/2

== system walkingRobotRL3D/Walking Robot (Angle based)/Dynamic model of antagonistic PAM actuators/Spring//Damping (Muscles 2)/Get_x2_hipD_pitch ==
  F1_hipD_pitch : Inport
  F2_hipD_pitch : Inport  Port=2
  S2_coef : Inport  Port=3
  Add : Sum  Inputs=-+-
  Constant : Constant  Value=tau
  Constant1 : Constant
  D_coef : Product
  Divide : Product  Inputs=*/
  Integrator : Integrator  InitialCondition=x20_hipD_pitch
  x./D : Product
  xS : Product
  x2_hipD_pitch : Outport
  wires:
  xS/1 -> Add/3
  Add/1 -> x./D/2
  F1_hipD_pitch/1 -> Add/1
  F2_hipD_pitch/1 -> Add/2
  Integrator/1 -> x2_hipD_pitch/1, xS/1
  S2_coef/1 -> D_coef/2, xS/2
  x./D/1 -> Integrator/1
  Constant/1 -> D_coef/1
  Divide/1 -> x./D/1
  Constant1/1 -> Divide/1
  D_coef/1 -> Divide/2

== system walkingRobotRL3D/Walking Robot (Angle based)/Dynamic model of antagonistic PAM actuators/Spring//Damping (Muscles 2)/Get_x2_hipD_roll ==
  F1_hipD_roll : Inport
  F2_hipD_roll : Inport  Port=2
  S2_coef : Inport  Port=3
  Add : Sum  Inputs=-+-
  Constant : Constant  Value=tau
  Constant1 : Constant
  D_coef : Product
  Divide : Product  Inputs=*/
  Integrator : Integrator  InitialCondition=x20_hipD_roll
  x./D : Product
  xS : Product
  x2_hipD_roll : Outport
  wires:
  xS/1 -> Add/3
  Add/1 -> x./D/2
  F1_hipD_roll/1 -> Add/1
  F2_hipD_roll/1 -> Add/2
  Integrator/1 -> x2_hipD_roll/1, xS/1
  S2_coef/1 -> D_coef/2, xS/2
  x./D/1 -> Integrator/1
  Constant/1 -> D_coef/1
  Divide/1 -> x./D/1
  Constant1/1 -> Divide/1
  D_coef/1 -> Divide/2

== system walkingRobotRL3D/Walking Robot (Angle based)/Dynamic model of antagonistic PAM actuators/Spring//Damping (Muscles 2)/Get_x2_hipI_pitch ==
  F1_hipI_pitch : Inport
  F2_hipI_pitch : Inport  Port=2
  S2_coef : Inport  Port=3
  Add : Sum  Inputs=-+-
  Constant : Constant  Value=tau
  Constant1 : Constant
  D_coef : Product
  Divide : Product  Inputs=*/
  Integrator : Integrator  InitialCondition=x20_hipI_pitch
  Relay : Relay  Commented=through  OnSwitchValue=28.12*muscle_nominal_length/100  OffSwitchValue=0  OnOutputValue=28.12*muscle_nominal_length/100
  x./D : Product
  xS : Product
  x2_hipI_pitch : Outport
  wires:
  xS/1 -> Add/3
  Add/1 -> x./D/2
  F1_hipI_pitch/1 -> Add/1
  F2_hipI_pitch/1 -> Add/2
  Integrator/1 -> Relay/1
  S2_coef/1 -> D_coef/2, xS/2
  x./D/1 -> Integrator/1
  Constant/1 -> D_coef/1
  Divide/1 -> x./D/1
  Constant1/1 -> Divide/1
  D_coef/1 -> Divide/2
  Relay/1 -> x2_hipI_pitch/1, xS/1

== system walkingRobotRL3D/Walking Robot (Angle based)/Dynamic model of antagonistic PAM actuators/Spring//Damping (Muscles 2)/Get_x2_hipI_roll ==
  F1_hipI_roll : Inport
  F2_hipI_roll : Inport  Port=2
  S2_coef : Inport  Port=3
  Add : Sum  Inputs=-+-
  Constant : Constant  Value=tau
  Constant1 : Constant
  D_coef : Product
  Divide : Product  Inputs=*/
  Integrator : Integrator  InitialCondition=x20_hipI_roll
  x./D : Product
  xS : Product
  x2_hipI_roll : Outport
  wires:
  xS/1 -> Add/3
  Add/1 -> x./D/2
  F1_hipI_roll/1 -> Add/1
  F2_hipI_roll/1 -> Add/2
  Integrator/1 -> x2_hipI_roll/1, xS/1
  S2_coef/1 -> D_coef/2, xS/2
  x./D/1 -> Integrator/1
  Constant/1 -> D_coef/1
  Divide/1 -> x./D/1
  Constant1/1 -> Divide/1
  D_coef/1 -> Divide/2

== system walkingRobotRL3D/Walking Robot (Angle based)/Dynamic model of antagonistic PAM actuators/Spring//Damping (Muscles 2)/Get_x2_kneeD ==
  F1_kneeD : Inport
  F2_kneeI : Inport  Port=2
  S2_coef : Inport  Port=3
  Add : Sum  Inputs=-+-
  Constant : Constant  Value=tau
  Constant1 : Constant
  D_coef : Product
  Divide : Product  Inputs=*/
  Integrator : Integrator  InitialCondition=x20_kneeD
  x./D : Product
  xS : Product
  x2_kneeD : Outport
  wires:
  xS/1 -> Add/3
  Add/1 -> x./D/2
  F1_kneeD/1 -> Add/1
  F2_kneeI/1 -> Add/2
  Integrator/1 -> x2_kneeD/1, xS/1
  S2_coef/1 -> D_coef/2, xS/2
  x./D/1 -> Integrator/1
  Constant/1 -> D_coef/1
  Divide/1 -> x./D/1
  Constant1/1 -> Divide/1
  D_coef/1 -> Divide/2

== system walkingRobotRL3D/Walking Robot (Angle based)/Dynamic model of antagonistic PAM actuators/Spring//Damping (Muscles 2)/Get_x2_kneeI ==
  F1_kneeI : Inport
  F2_kneeI : Inport  Port=2
  S2_coef : Inport  Port=3
  Add : Sum  Inputs=++-
  Constant : Constant  Value=tau
  Constant1 : Constant
  D_coef : Product
  Divide : Product  Inputs=*/
  Integrator : Integrator  InitialCondition=x20_kneeI
  x./D : Product
  xS : Product
  x2_kneeI : Outport
  wires:
  xS/1 -> Add/3
  Add/1 -> x./D/2
  F1_kneeI/1 -> Add/1
  F2_kneeI/1 -> Add/2
  Integrator/1 -> x2_kneeI/1, xS/1
  S2_coef/1 -> D_coef/2, xS/2
  x./D/1 -> Integrator/1
  Constant/1 -> D_coef/1
  Divide/1 -> x./D/1
  Constant1/1 -> Divide/1
  D_coef/1 -> Divide/2

== system walkingRobotRL3D/Walking Robot (Angle based)/Dynamic model of antagonistic PAM actuators/Spring//Damping (Muscles 2)/Getxmax2 ==
  P2 : Inport
  Get_delta_xmax1 : Subsystem
  delta_xmax_muscles2 : Outport
  delta_xmax_muscles2_per : Outport  Port=2
  wires:
  P2/1 -> Get_delta_xmax1/1(P2)
  Get_delta_xmax1/1(delta_xmax_muscles2) -> delta_xmax_muscles2/1
  Get_delta_xmax1/2(delta_xmax_muscles2_per) -> delta_xmax_muscles2_per/1

== system walkingRobotRL3D/Walking Robot1/Dynamic model of antagonistic PAM actuators/Spring//Damping (Muscles 1)/Get_x1_ankleD_pitch ==
  F1_ankleD_pitchl : Inport
  F2_ankleD_pitch : Inport  Port=2
  S_coef : Inport  Port=3
  Add : Sum  Inputs=+--
  Constant : Constant  Value=tau
  Constant1 : Constant
  Constant2 : Constant  Commented=on  Value=-3.9322
  D_coef : Product
  Divide : Product  Inputs=*/
  IC : InitialCondition  Commented=through  Value=-3.9322
  Integrator : Integrator  InitialCondition=x10_ankleD_pitch
  x./D : Product
  xS : Product
  x1_ankleD_pitch : Outport
  wires:
  xS/1 -> Add/3
  x./D/1 -> Integrator/1
  Constant/1 -> D_coef/1
  Divide/1 -> x./D/1
  Constant1/1 -> Divide/1
  D_coef/1 -> Divide/2
  Integrator/1 -> x1_ankleD_pitch/1, xS/1
  IC/1 -> xS/2, D_coef/2
  F1_ankleD_pitchl/1 -> Add/1
  F2_ankleD_pitch/1 -> Add/2
  S_coef/1 -> IC/1
  Add/1 -> x./D/2

== system walkingRobotRL3D/Walking Robot1/Dynamic model of antagonistic PAM actuators/Spring//Damping (Muscles 1)/Get_x1_ankleD_roll ==
  F1_ankleD_roll : Inport
  F2_ankleD_roll : Inport  Port=2
  S_coef : Inport  Port=3
  Add : Sum  Inputs=+--
  Constant : Constant  Value=tau
  Constant1 : Constant
  Constant2 : Constant  Commented=on  Value=-3.9322
  D_coef : Product
  Divide : Product  Inputs=*/
  IC : InitialCondition  Commented=through  Value=-3.9322
  Integrator : Integrator  InitialCondition=x10_ankleD_roll
  x./D : Product
  xS : Product
  x1_ankleD_roll : Outport
  wires:
  xS/1 -> Add/3
  x./D/1 -> Integrator/1
  Constant/1 -> D_coef/1
  Divide/1 -> x./D/1
  Constant1/1 -> Divide/1
  D_coef/1 -> Divide/2
  Integrator/1 -> x1_ankleD_roll/1, xS/1
  IC/1 -> xS/2, D_coef/2
  F1_ankleD_roll/1 -> Add/1
  F2_ankleD_roll/1 -> Add/2
  S_coef/1 -> IC/1
  Add/1 -> x./D/2

== system walkingRobotRL3D/Walking Robot1/Dynamic model of antagonistic PAM actuators/Spring//Damping (Muscles 1)/Get_x1_ankleI_pitch ==
  F1_ankleI_pitch : Inport
  F2_ankleI_pitch : Inport  Port=2
  S_coef : Inport  Port=3
  Add : Sum  Inputs=+--
  Constant : Constant  Value=tau
  Constant1 : Constant
  D_coef : Product
  Divide : Product  Inputs=*/
  Integrator : Integrator  InitialCondition=x10_ankleI_pitch
  x./D : Product
  xS : Product
  x1_ankleI_pitch : Outport
  wires:
  xS/1 -> Add/3
  Add/1 -> x./D/2
  F1_ankleI_pitch/1 -> Add/1
  F2_ankleI_pitch/1 -> Add/2
  Integrator/1 -> x1_ankleI_pitch/1, xS/1
  S_coef/1 -> D_coef/2, xS/2
  x./D/1 -> Integrator/1
  Constant/1 -> D_coef/1
  Divide/1 -> x./D/1
  Constant1/1 -> Divide/1
  D_coef/1 -> Divide/2

== system walkingRobotRL3D/Walking Robot1/Dynamic model of antagonistic PAM actuators/Spring//Damping (Muscles 1)/Get_x1_ankleI_roll ==
  F1_ankleI_roll : Inport
  F2_ankleI_roll : Inport  Port=2
  S_coef : Inport  Port=3
  Add : Sum  Inputs=+--
  Constant : Constant  Value=tau
  Constant1 : Constant
  D_coef : Product
  Divide : Product  Inputs=*/
  Integrator : Integrator  InitialCondition=x10_ankleI_roll
  x./D : Product
  xS : Product
  x1_ankleI_roll : Outport
  wires:
  xS/1 -> Add/3
  Add/1 -> x./D/2
  F1_ankleI_roll/1 -> Add/1
  F2_ankleI_roll/1 -> Add/2
  Integrator/1 -> x1_ankleI_roll/1, xS/1
  S_coef/1 -> D_coef/2, xS/2
  x./D/1 -> Integrator/1
  Constant/1 -> D_coef/1
  Divide/1 -> x./D/1
  Constant1/1 -> Divide/1
  D_coef/1 -> Divide/2

== system walkingRobotRL3D/Walking Robot1/Dynamic model of antagonistic PAM actuators/Spring//Damping (Muscles 1)/Get_x1_hipD_pitch ==
  F1_hipD_pitch : Inport
  F2_hipD_pitch : Inport  Port=2
  S_coef : Inport  Port=3
  Add : Sum  Inputs=+--
  Constant : Constant  Value=tau
  Constant1 : Constant
  D_coef : Product
  Divide : Product  Inputs=*/
  Integrator : Integrator  InitialCondition=x10_hipD_pitch
  x./D : Product
  xS : Product
  x1_hipD_pitch : Outport
  wires:
  xS/1 -> Add/3
  Add/1 -> x./D/2
  F1_hipD_pitch/1 -> Add/1
  F2_hipD_pitch/1 -> Add/2
  Integrator/1 -> x1_hipD_pitch/1, xS/1
  S_coef/1 -> D_coef/2, xS/2
  x./D/1 -> Integrator/1
  Constant/1 -> D_coef/1
  Divide/1 -> x./D/1
  Constant1/1 -> Divide/1
  D_coef/1 -> Divide/2

== system walkingRobotRL3D/Walking Robot1/Dynamic model of antagonistic PAM actuators/Spring//Damping (Muscles 1)/Get_x1_hipD_roll ==
  F1_hipD_roll : Inport
  F2_hipD_roll : Inport  Port=2
  S_coef : Inport  Port=3
  Add : Sum  Inputs=+--
  Constant : Constant  Value=tau
  Constant1 : Constant
  D_coef : Product
  Divide : Product  Inputs=*/
  Integrator : Integrator  InitialCondition=x10_hipD_roll
  x./D : Product
  xS : Product
  x1_hipD_roll : Outport
  wires:
  xS/1 -> Add/3
  Add/1 -> x./D/2
  F1_hipD_roll/1 -> Add/1
  F2_hipD_roll/1 -> Add/2
  Integrator/1 -> x1_hipD_roll/1, xS/1
  S_coef/1 -> D_coef/2, xS/2
  x./D/1 -> Integrator/1
  Constant/1 -> D_coef/1
  Divide/1 -> x./D/1
  Constant1/1 -> Divide/1
  D_coef/1 -> Divide/2

== system walkingRobotRL3D/Walking Robot1/Dynamic model of antagonistic PAM actuators/Spring//Damping (Muscles 1)/Get_x1_hipI_pitch ==
  F1_hipI_pitch : Inport
  F2_hipI_pitch : Inport  Port=2
  S_coef : Inport  Port=3
  Add : Sum  Inputs=+--
  Constant : Constant  Value=tau
  Constant1 : Constant
  D_coef : Product
  Divide : Product  Inputs=*/
  Integrator : Integrator  InitialCondition=x10_hipI_pitch
  x./D : Product
  xS : Product
  x1_hipI_pitch : Outport
  wires:
  xS/1 -> Add/3
  Add/1 -> x./D/2
  F1_hipI_pitch/1 -> Add/1
  F2_hipI_pitch/1 -> Add/2
  Integrator/1 -> x1_hipI_pitch/1, xS/1
  S_coef/1 -> D_coef/2, xS/2
  x./D/1 -> Integrator/1
  Constant/1 -> D_coef/1
  Divide/1 -> x./D/1
  Constant1/1 -> Divide/1
  D_coef/1 -> Divide/2

== system walkingRobotRL3D/Walking Robot1/Dynamic model of antagonistic PAM actuators/Spring//Damping (Muscles 1)/Get_x1_hipI_roll ==
  F1_hipI_roll : Inport
  F2_hipI_roll : Inport  Port=2
  S_coef : Inport  Port=3
  Add : Sum  Inputs=+--
  Constant : Constant  Value=tau
  Constant1 : Constant
  D_coef : Product
  Divide : Product  Inputs=*/
  Integrator : Integrator  InitialCondition=x10_hipI_roll
  x./D : Product
  xS : Product
  x1_hipI_roll : Outport
  wires:
  xS/1 -> Add/3
  Add/1 -> x./D/2
  F1_hipI_roll/1 -> Add/1
  F2_hipI_roll/1 -> Add/2
  Integrator/1 -> x1_hipI_roll/1, xS/1
  S_coef/1 -> D_coef/2, xS/2
  x./D/1 -> Integrator/1
  Constant/1 -> D_coef/1
  Divide/1 -> x./D/1
  Constant1/1 -> Divide/1
  D_coef/1 -> Divide/2

== system walkingRobotRL3D/Walking Robot1/Dynamic model of antagonistic PAM actuators/Spring//Damping (Muscles 1)/Get_x1_kneeD_1 ==
  F1_kneeD : Inport
  F2_kneeD : Inport  Port=2
  S_coef : Inport  Port=3
  Add : Sum  Inputs=+--
  Constant : Constant  Value=tau
  Constant1 : Constant
  D_coef : Product
  Divide : Product  Inputs=*/
  Integrator : Integrator  InitialCondition=x10_kneeD
  x./D : Product
  xS : Product
  x1_kneeD : Outport
  wires:
  xS/1 -> Add/3
  Add/1 -> x./D/2
  F1_kneeD/1 -> Add/1
  F2_kneeD/1 -> Add/2
  Integrator/1 -> x1_kneeD/1, xS/1
  S_coef/1 -> D_coef/2, xS/2
  x./D/1 -> Integrator/1
  Constant/1 -> D_coef/1
  Divide/1 -> x./D/1
  Constant1/1 -> Divide/1
  D_coef/1 -> Divide/2

== system walkingRobotRL3D/Walking Robot1/Dynamic model of antagonistic PAM actuators/Spring//Damping (Muscles 1)/Get_x1_kneeI ==
  F1_kneeI : Inport
  F2_kneeI : Inport  Port=2
  S_coef : Inport  Port=3
  Add : Sum  Inputs=+--
  Constant : Constant  Value=tau
  Constant1 : Constant
  D_coef : Product
  Divide : Product  Inputs=*/
  Integrator : Integrator  InitialCondition=x10_kneeI
  x./D : Product
  xS : Product
  x1_kneeI : Outport
  wires:
  xS/1 -> Add/3
  Add/1 -> x./D/2
  F1_kneeI/1 -> Add/1
  F2_kneeI/1 -> Add/2
  Integrator/1 -> x1_kneeI/1, xS/1
  S_coef/1 -> D_coef/2, xS/2
  x./D/1 -> Integrator/1
  Constant/1 -> D_coef/1
  Divide/1 -> x./D/1
  Constant1/1 -> Divide/1
  D_coef/1 -> Divide/2

== system walkingRobotRL3D/Walking Robot1/Dynamic model of antagonistic PAM actuators/Spring//Damping (Muscles 1)/Getxmax1 ==
  P1 : Inport
  Bar->kPa : Product
  Constant : Constant  Value=100
  Demux : Demux  Outputs=10
  Mux : Mux  Inputs=10
  getMaxStroke : MATLAB Function  TreatAsAtomicUnit=on
  getMaxStroke1 : MATLAB Function  TreatAsAtomicUnit=on
  getMaxStroke2 : MATLAB Function  TreatAsAtomicUnit=on
  getMaxStroke3 : MATLAB Function  TreatAsAtomicUnit=on
  getMaxStroke4 : MATLAB Function  TreatAsAtomicUnit=on
  getMaxStroke5 : MATLAB Function  TreatAsAtomicUnit=on
  getMaxStroke6 : MATLAB Function  TreatAsAtomicUnit=on
  getMaxStroke7 : MATLAB Function  TreatAsAtomicUnit=on
  getMaxStroke8 : MATLAB Function  TreatAsAtomicUnit=on
  getMaxStroke9 : MATLAB Function  TreatAsAtomicUnit=on
  xmax_muscles1 : Outport
  wires:
  Mux/1 -> xmax_muscles1/1
  getMaxStroke/1(x_max1) -> Mux/1
  P1/1 -> Bar->kPa/2
  Bar->kPa/1 -> Demux/1
  Constant/1 -> Bar->kPa/1
  Demux/1 -> getMaxStroke/1(P1)
  Demux/2 -> getMaxStroke1/1(P1)
  Demux/3 -> getMaxStroke2/1(P1)
  Demux/4 -> getMaxStroke3/1(P1)
  Demux/5 -> getMaxStroke4/1(P1)
  Demux/6 -> getMaxStroke5/1(P1)
  Demux/7 -> getMaxStroke6/1(P1)
  Demux/8 -> getMaxStroke7/1(P1)
  Demux/9 -> getMaxStroke8/1(P1)
  getMaxStroke1/1(x_max1) -> Mux/2
  getMaxStroke2/1(x_max1) -> Mux/3
  getMaxStroke3/1(x_max1) -> Mux/4
  getMaxStroke4/1(x_max1) -> Mux/5
  getMaxStroke5/1(x_max1) -> Mux/6
  getMaxStroke6/1(x_max1) -> Mux/7
  getMaxStroke7/1(x_max1) -> Mux/8
  getMaxStroke8/1(x_max1) -> Mux/9
  Demux/10 -> getMaxStroke9/1(P1)
  getMaxStroke9/1(x_max1) -> Mux/10

== system walkingRobotRL3D/Walking Robot1/Dynamic model of antagonistic PAM actuators/Spring//Damping (Muscles 2)/Get_x2_ankleD_pitch ==
  F1_ankleD_pitch : Inport
  F2_ankleD_pitch : Inport  Port=2
  S2_coef : Inport  Port=3
  Add : Sum  Inputs=-+-
  Constant : Constant  Value=tau
  Constant1 : Constant
  Constant2 : Constant  Commented=on  Value=3.9338
  D_coef : Product
  Divide : Product  Inputs=*/
  IC : InitialCondition  Commented=through  Value=3.9338
  Integrator : Integrator  InitialCondition=x20_ankleD_pitch
  x./D : Product
  xS : Product
  x2_ankleD_pitch : Outport
  wires:
  xS/1 -> Add/3
  Add/1 -> x./D/2
  F1_ankleD_pitch/1 -> Add/1
  F2_ankleD_pitch/1 -> Add/2
  Integrator/1 -> x2_ankleD_pitch/1, xS/1
  x./D/1 -> Integrator/1
  Constant/1 -> D_coef/1
  Divide/1 -> x./D/1
  Constant1/1 -> Divide/1
  IC/1 -> D_coef/2, xS/2
  D_coef/1 -> Divide/2
  S2_coef/1 -> IC/1

== system walkingRobotRL3D/Walking Robot1/Dynamic model of antagonistic PAM actuators/Spring//Damping (Muscles 2)/Get_x2_ankleD_roll ==
  F1_ankleD_roll : Inport
  F2_ankleD_roll : Inport  Port=2
  S2_coef : Inport  Port=3
  Add : Sum  Inputs=-+-
  Constant : Constant  Value=tau
  Constant1 : Constant
  Constant2 : Constant  Commented=on  Value=3.9338
  D_coef : Product
  Divide : Product  Inputs=*/
  IC : InitialCondition  Commented=through  Value=3.9338
  Integrator : Integrator  InitialCondition=x20_ankleD_roll
  x./D : Product
  xS : Product
  x2_ankleD_roll : Outport
  wires:
  xS/1 -> Add/3
  Add/1 -> x./D/2
  F1_ankleD_roll/1 -> Add/1
  F2_ankleD_roll/1 -> Add/2
  Integrator/1 -> x2_ankleD_roll/1, xS/1
  x./D/1 -> Integrator/1
  Constant/1 -> D_coef/1
  Divide/1 -> x./D/1
  Constant1/1 -> Divide/1
  IC/1 -> D_coef/2, xS/2
  D_coef/1 -> Divide/2
  S2_coef/1 -> IC/1

== system walkingRobotRL3D/Walking Robot1/Dynamic model of antagonistic PAM actuators/Spring//Damping (Muscles 2)/Get_x2_ankleI_pitch ==
  F1_ankleI_pitch : Inport
  F2_ankleI_pitch : Inport  Port=2
  S2_coef : Inport  Port=3
  Add : Sum  Inputs=-+-
  Constant : Constant  Value=tau
  Constant1 : Constant
  D_coef : Product
  Divide : Product  Inputs=*/
  Integrator : Integrator  InitialCondition=x20_ankleI_pitch
  x./D : Product
  xS : Product
  x2_ankleI_pitch : Outport
  wires:
  xS/1 -> Add/3
  Add/1 -> x./D/2
  F1_ankleI_pitch/1 -> Add/1
  F2_ankleI_pitch/1 -> Add/2
  Integrator/1 -> x2_ankleI_pitch/1, xS/1
  S2_coef/1 -> D_coef/2, xS/2
  x./D/1 -> Integrator/1
  Constant/1 -> D_coef/1
  Divide/1 -> x./D/1
  Constant1/1 -> Divide/1
  D_coef/1 -> Divide/2

== system walkingRobotRL3D/Walking Robot1/Dynamic model of antagonistic PAM actuators/Spring//Damping (Muscles 2)/Get_x2_ankleI_roll ==
  F1_ankleI_roll : Inport
  F2_ankleI_roll : Inport  Port=2
  S2_coef : Inport  Port=3
  Add : Sum  Inputs=-+-
  Constant : Constant  Value=tau
  Constant1 : Constant
  D_coef : Product
  Divide : Product  Inputs=*/
  Integrator : Integrator  InitialCondition=x20_ankleI_roll
  x./D : Product
  xS : Product
  x2_ankleI_roll : Outport
  wires:
  xS/1 -> Add/3
  Add/1 -> x./D/2
  F1_ankleI_roll/1 -> Add/1
  F2_ankleI_roll/1 -> Add/2
  Integrator/1 -> x2_ankleI_roll/1, xS/1
  S2_coef/1 -> D_coef/2, xS/2
  x./D/1 -> Integrator/1
  Constant/1 -> D_coef/1
  Divide/1 -> x./D/1
  Constant1/1 -> Divide/1
  D_coef/1 -> Divide/2

== system walkingRobotRL3D/Walking Robot1/Dynamic model of antagonistic PAM actuators/Spring//Damping (Muscles 2)/Get_x2_hipD_pitch ==
  F1_hipD_pitch : Inport
  F2_hipD_pitch : Inport  Port=2
  S2_coef : Inport  Port=3
  Add : Sum  Inputs=-+-
  Constant : Constant  Value=tau
  Constant1 : Constant
  D_coef : Product
  Divide : Product  Inputs=*/
  Integrator : Integrator  InitialCondition=x20_hipD_pitch
  x./D : Product
  xS : Product
  x2_hipD_pitch : Outport
  wires:
  xS/1 -> Add/3
  Add/1 -> x./D/2
  F1_hipD_pitch/1 -> Add/1
  F2_hipD_pitch/1 -> Add/2
  Integrator/1 -> x2_hipD_pitch/1, xS/1
  S2_coef/1 -> D_coef/2, xS/2
  x./D/1 -> Integrator/1
  Constant/1 -> D_coef/1
  Divide/1 -> x./D/1
  Constant1/1 -> Divide/1
  D_coef/1 -> Divide/2

== system walkingRobotRL3D/Walking Robot1/Dynamic model of antagonistic PAM actuators/Spring//Damping (Muscles 2)/Get_x2_hipD_roll ==
  F1_hipD_roll : Inport
  F2_hipD_roll : Inport  Port=2
  S2_coef : Inport  Port=3
  Add : Sum  Inputs=-+-
  Constant : Constant  Value=tau
  Constant1 : Constant
  D_coef : Product
  Divide : Product  Inputs=*/
  Integrator : Integrator  InitialCondition=x20_hipD_roll
  x./D : Product
  xS : Product
  x2_hipD_roll : Outport
  wires:
  xS/1 -> Add/3
  Add/1 -> x./D/2
  F1_hipD_roll/1 -> Add/1
  F2_hipD_roll/1 -> Add/2
  Integrator/1 -> x2_hipD_roll/1, xS/1
  S2_coef/1 -> D_coef/2, xS/2
  x./D/1 -> Integrator/1
  Constant/1 -> D_coef/1
  Divide/1 -> x./D/1
  Constant1/1 -> Divide/1
  D_coef/1 -> Divide/2

== system walkingRobotRL3D/Walking Robot1/Dynamic model of antagonistic PAM actuators/Spring//Damping (Muscles 2)/Get_x2_hipI_pitch ==
  F1_hipI_pitch : Inport
  F2_hipI_pitch : Inport  Port=2
  S2_coef : Inport  Port=3
  Add : Sum  Inputs=-+-
  Constant : Constant  Value=tau
  Constant1 : Constant
  D_coef : Product
  Divide : Product  Inputs=*/
  Integrator : Integrator  InitialCondition=x20_hipI_pitch
  x./D : Product
  xS : Product
  x2_hipI_pitch : Outport
  wires:
  xS/1 -> Add/3
  Add/1 -> x./D/2
  F1_hipI_pitch/1 -> Add/1
  F2_hipI_pitch/1 -> Add/2
  Integrator/1 -> x2_hipI_pitch/1, xS/1
  S2_coef/1 -> D_coef/2, xS/2
  x./D/1 -> Integrator/1
  Constant/1 -> D_coef/1
  Divide/1 -> x./D/1
  Constant1/1 -> Divide/1
  D_coef/1 -> Divide/2

== system walkingRobotRL3D/Walking Robot1/Dynamic model of antagonistic PAM actuators/Spring//Damping (Muscles 2)/Get_x2_hipI_roll ==
  F1_hipI_roll : Inport
  F2_hipI_roll : Inport  Port=2
  S2_coef : Inport  Port=3
  Add : Sum  Inputs=-+-
  Constant : Constant  Value=tau
  Constant1 : Constant
  D_coef : Product
  Divide : Product  Inputs=*/
  Integrator : Integrator  InitialCondition=x20_hipI_roll
  x./D : Product
  xS : Product
  x2_hipI_roll : Outport
  wires:
  xS/1 -> Add/3
  Add/1 -> x./D/2
  F1_hipI_roll/1 -> Add/1
  F2_hipI_roll/1 -> Add/2
  Integrator/1 -> x2_hipI_roll/1, xS/1
  S2_coef/1 -> D_coef/2, xS/2
  x./D/1 -> Integrator/1
  Constant/1 -> D_coef/1
  Divide/1 -> x./D/1
  Constant1/1 -> Divide/1
  D_coef/1 -> Divide/2

== system walkingRobotRL3D/Walking Robot1/Dynamic model of antagonistic PAM actuators/Spring//Damping (Muscles 2)/Get_x2_kneeD ==
  F1_kneeD : Inport
  F2_kneeI : Inport  Port=2
  S2_coef : Inport  Port=3
  Add : Sum  Inputs=-+-
  Constant : Constant  Value=tau
  Constant1 : Constant
  D_coef : Product
  Divide : Product  Inputs=*/
  Integrator : Integrator  InitialCondition=x20_kneeD
  x./D : Product
  xS : Product
  x2_kneeD : Outport
  wires:
  xS/1 -> Add/3
  Add/1 -> x./D/2
  F1_kneeD/1 -> Add/1
  F2_kneeI/1 -> Add/2
  Integrator/1 -> x2_kneeD/1, xS/1
  S2_coef/1 -> D_coef/2, xS/2
  x./D/1 -> Integrator/1
  Constant/1 -> D_coef/1
  Divide/1 -> x./D/1
  Constant1/1 -> Divide/1
  D_coef/1 -> Divide/2

== system walkingRobotRL3D/Walking Robot1/Dynamic model of antagonistic PAM actuators/Spring//Damping (Muscles 2)/Get_x2_kneeI ==
  F1_kneeI : Inport
  F2_kneeI : Inport  Port=2
  S2_coef : Inport  Port=3
  Add : Sum  Inputs=-+-
  Constant : Constant  Value=tau
  Constant1 : Constant
  D_coef : Product
  Divide : Product  Inputs=*/
  Integrator : Integrator  InitialCondition=x20_kneeI
  x./D : Product
  xS : Product
  x2_kneeI : Outport
  wires:
  xS/1 -> Add/3
  Add/1 -> x./D/2
  F1_kneeI/1 -> Add/1
  F2_kneeI/1 -> Add/2
  Integrator/1 -> x2_kneeI/1, xS/1
  S2_coef/1 -> D_coef/2, xS/2
  x./D/1 -> Integrator/1
  Constant/1 -> D_coef/1
  Divide/1 -> x./D/1
  Constant1/1 -> Divide/1
  D_coef/1 -> Divide/2
